simulink model "s_spg_pp"  (Simulink 10.3)
settings: Solver=ode4  StartTime=0.0  StopTime=10  FixedStep=0.002  RelTol=1e-3  AbsTol=1e-6  EnableMultiTasking=on
values from neighbouring files (symbols this model uses):
  K = [ 0 0 0 0 ]    [setup_ip02_spg.m]
  wcf = 2 * pi * 10    (= 62.8318530718)    [setup_ip02_spg.m]
  X0 = [ 0; X0(2); 0; 0 ]    [setup_ip02_spg.m]
  zetaf = 0.9    [setup_ip02_spg.m]
undefined symbols (not defined in the file or in its folder): A, B, C, D, Lp, VMAX_AMP
libraries: simulink_extras x1
settings Model: Creator=MLevis  LastModifiedBy=MLevis  ExtModeTrigDuration=5000  ExtModeArmWhenConnect=off
settings SolverCC: AutoScaleAbsTol=off  PositivePriorityOrder=on
settings OptimizationCC: BooleanDataType=off  OptimizeBlockIOStorage=off  BufferReuse=off  ExpressionFolding=off  LocalBlockOutputs=off  InitFltsAndDblsToZero=on  LifeSpan=auto
settings DebuggingCC: SaveWithParameterizedLinksMsg=none  SignalResolutionControl=TryResolveAllWithWarning  MultiTaskDSMMsg=warning  MultiTaskCondExecSysMsg=none
settings HardwareCC: ProdLargestAtomicFloat=Float  ProdIntDivRoundTo=Zero  ProdEndianess=LittleEndian  ProdHWDeviceType=Intel->x86-32 (Windows32)
settings RTWCC: Description=QUARC Win32 Target Using Toolchain  SystemTargetFile=quarc_windows.tlc  TemplateMakefile=quarc_default_tmf  Toolchain=QUARC windows | nmake (64-bit Windows)  BuildConfiguration=Faster Runs
settings STFCustomTargetCC: ConcurrentExecutionCompliant=on  UseToolchainInfoCompliant=on  SystemTargetFile=quarc_windows.tlc
settings GRTTargetCC: ParMdlRefBuildCompliant=off  CompOptLevelCompliant=off  MatFileLogging=off  CPPClassGenCompliant=off  ExtMode=on  ExtModeMexFile=quarc_comm

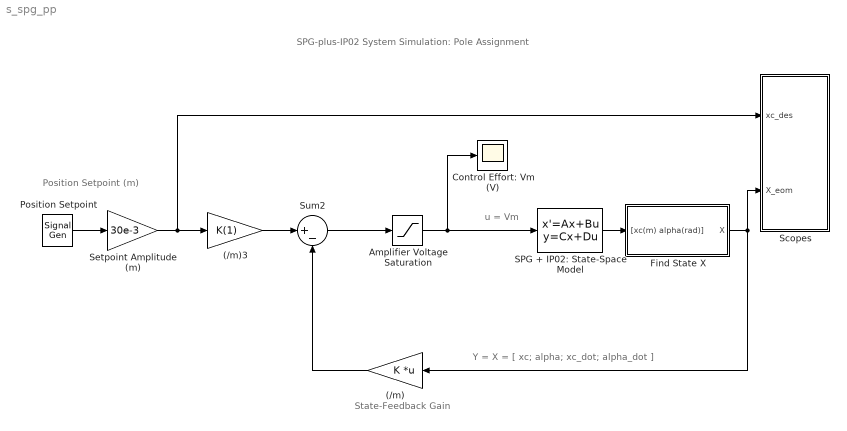
== system s_spg_pp ==
  note: u = Vm
  note: Y = X = [ xc; alpha; xc_dot; alpha_dot ]
  note: State-Feedback Gain
  note: Position Setpoint (m)
  note: SPG-plus-IP02 System Simulation:
      | Pole Assignment
  (/m) : Gain  Gain=K  Multiplication=Matrix(K*u)  SaturateOnIntegerOverflow=on  OutDataTypeStr=Inherit: Same as input  ParamDataTypeStr=Inherit: Same as input
  (/m)3 : Gain  Gain=K(1)  SaturateOnIntegerOverflow=on  OutDataTypeStr=Inherit: Same as input  ParamDataTypeStr=Inherit: Same as input
  Amplifier Voltage Saturation : Saturate  UpperLimit=VMAX_AMP  LowerLimit=- VMAX_AMP
  Control Effort: Vm (V) : Scope
  Find State X : Subsystem
  Position Setpoint : SignalGenerator  WaveForm=square  Frequency=0.1
  SPG + IP02: State-Space Model : StateSpace  A=A  B=B  C=C  D=D  InitialCondition=X0
  Scopes : Subsystem
  Setpoint Amplitude (m) : Gain  Gain=30e-3  SaturateOnIntegerOverflow=on  OutDataTypeStr=Inherit: Same as input  ParamDataTypeStr=Inherit: Same as input
  Sum2 : Sum  Inputs=|+-  InputSameDT=on  SaturateOnIntegerOverflow=on  OutDataTypeStr=Inherit: Same as first input
  wires:
  Amplifier Voltage Saturation/1 -> Control Effort: Vm (V)/1, SPG + IP02: State-Space Model/1
  (/m)3/1 -> Sum2/1
  Setpoint Amplitude (m)/1 -> Scopes/1(xc_des), (/m)3/1
  Position Setpoint/1 -> Setpoint Amplitude (m)/1
  (/m)/1 -> Sum2/2
  Sum2/1 -> Amplifier Voltage Saturation/1
  SPG + IP02: State-Space Model/1 -> Find State X/1("[xc(m) alpha(rad)]")
  Find State X/1(X) -> Scopes/2(X_eom), (/m)/1

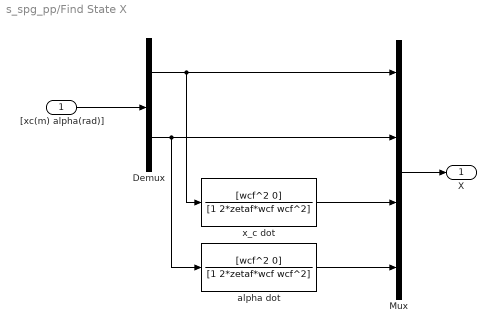
== system s_spg_pp/Find State X ==
  "[xc(m) alpha(rad)]" : Inport
  Demux : Demux  Outputs=2
  Mux : Mux
  alpha dot : TransferFcn  Numerator=[wcf^2 0]  Denominator=[1 2*zetaf*wcf wcf^2]
  x_c dot : TransferFcn  Numerator=[wcf^2 0]  Denominator=[1 2*zetaf*wcf wcf^2]
  X : Outport
  wires:
  Mux/1 -> X/1
  x_c dot/1 -> Mux/3
  alpha dot/1 -> Mux/4
  "[xc(m) alpha(rad)]"/1 -> Demux/1
  Demux/1 -> Mux/1, x_c dot/1
  Demux/2 -> Mux/2, alpha dot/1

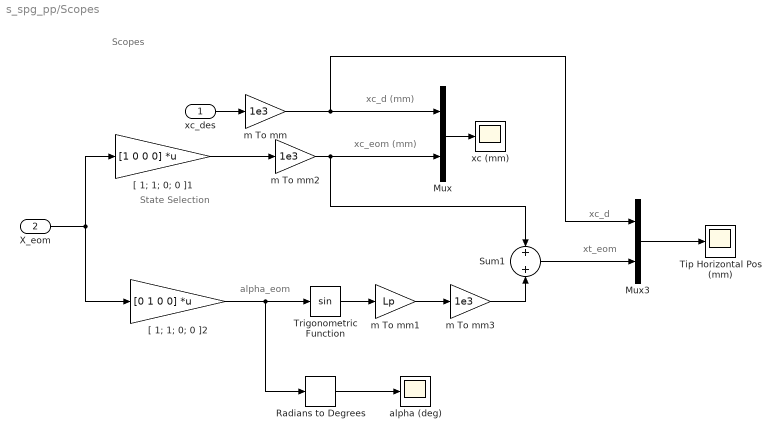
== system s_spg_pp/Scopes ==
  note: Scopes
  note: xc_d (mm)
  note: alpha_eom
  note: State Selection
  note: xc_eom (mm)
  note: xc_d
  note: xt_eom
  xc_des : Inport
  X_eom : Inport  Port=2
  Mux : Mux  Inputs=2
  Mux3 : Mux  Inputs=2
  Radians to Degrees : simulink_extras/Transformations/Radians to Degrees
  Sum1 : Sum  Inputs=+|+  InputSameDT=on  SaturateOnIntegerOverflow=on  OutDataTypeStr=Inherit: Same as first input
  Tip Horizontal Pos (mm) : Scope
  Trigonometric Function : Trigonometry
  "[ 1; 1; 0; 0 ]1" : Gain  Gain=[1 0 0 0]  Multiplication=Matrix(K*u)  SaturateOnIntegerOverflow=on  OutDataTypeStr=Inherit: Same as input  ParamDataTypeStr=Inherit: Same as input
  "[ 1; 1; 0; 0 ]2" : Gain  Gain=[0 1 0 0]  Multiplication=Matrix(K*u)  SaturateOnIntegerOverflow=on  OutDataTypeStr=Inherit: Same as input  ParamDataTypeStr=Inherit: Same as input
  alpha (deg) : Scope
  m To mm : Gain  Gain=1e3  SaturateOnIntegerOverflow=on  OutDataTypeStr=Inherit: Same as input  ParamDataTypeStr=Inherit: Same as input
  m To mm1 : Gain  Gain=Lp  SaturateOnIntegerOverflow=on  OutDataTypeStr=Inherit: Same as input  ParamDataTypeStr=Inherit: Same as input
  m To mm2 : Gain  Gain=1e3  SaturateOnIntegerOverflow=on  OutDataTypeStr=Inherit: Same as input  ParamDataTypeStr=Inherit: Same as input
  m To mm3 : Gain  Gain=1e3  SaturateOnIntegerOverflow=on  OutDataTypeStr=Inherit: Same as input  ParamDataTypeStr=Inherit: Same as input
  xc (mm) : Scope
  wires:
  "[ 1; 1; 0; 0 ]2"/1 -> Radians to Degrees/1, Trigonometric Function/1
  X_eom/1 -> "[ 1; 1; 0; 0 ]2"/1, "[ 1; 1; 0; 0 ]1"/1
  xc_des/1 -> m To mm/1
  "[ 1; 1; 0; 0 ]1"/1 -> m To mm2/1
  Mux/1 -> xc (mm)/1
  m To mm1/1 -> m To mm3/1
  Trigonometric Function/1 -> m To mm1/1
  m To mm3/1 -> Sum1/2
  Radians to Degrees/1 -> alpha (deg)/1
  Mux3/1 -> Tip Horizontal Pos (mm)/1
  Sum1/1 -> Mux3/2
  m To mm/1 -> Mux/1, Mux3/1
  m To mm2/1 -> Mux/2, Sum1/1
